simulink model "Motor_La"  (Simulink 7.9)
settings: Solver=ode45  StartTime=0.0  StopTime=0.2  MaxStep=0.0000008  RelTol=1e-8
values from neighbouring files (symbols this model uses):
  J_ges = Jm+Jc/i_getr^2    (= 1.07037741047e-06)    [Sim_Kinematik_Modelle.m]    (also in Tol_Kinematik_Modell.m = Jm+Jc/i_getr^2)
  La = 0*1.792e-3    (= 0)    [DC_Motor_RI_Comp.m]    (also in Sim_Kinematik_Modelle.m = 0.0067; Tol_Kinematik_Modell.m = rnd_vect(n_s,'normal',[La_nom La_tol/3]))
  M_motor = 0.8*M_Load    (= 0.000824029771398)    [DC_Motor_RI_Comp.m]    (also in Sim_Kinematik_Modelle.m = -0.00561973731383; Tol_Kinematik_Modell.m = M_last./(i_getr.*eta_getr))
  Mo = Io*Psi    (= 0.000558650326277)    [DC_Motor_RI_Comp.m]    (also in Sim_Kinematik_Modelle.m = 0.00152232213911; Tol_Kinematik_Modell.m = Io.*Psi)
  Psi = 1/Ispez    (= 0.0159159637116)    [DC_Motor_RI_Comp.m]    (also in Sim_Kinematik_Modelle.m = 0.0173484004456; Tol_Kinematik_Modell.m = Psi_20*(1+Kemf*(T(T_N)-20)))
  Ra = 6.7    [DC_Motor_RI_Comp.m]    (also in Sim_Kinematik_Modelle.m = 5.1322; Tol_Kinematik_Modell.m = Ra_20*(1+Kr*(T(T_N)-20)))
  T_on = linspace(0,0.05,800)    [DC_Motor_RI_Comp.m]    (also in Sim_Kinematik_Modelle.m; Tol_Kinematik_Modell.m = rnd_vect(n_s,'normal',[T_on_nom T_on_tol/3]))
  U_max = U_max_w(i_U)    [DC_Motor_RI_Comp.m]    (also in Sim_Kinematik_Modelle.m; Tol_Kinematik_Modell.m = rnd_vect(n_s,'normal',[U_max_nom U_max_tol/3]))
settings Model: Creator=dep02378  LastModifiedBy=dep02378
settings OptimizationCC: InitFltsAndDblsToZero=on
settings DebuggingCC: FcnCallInpInsideContextMsg=Use local settings  StrictBusMsg=Warning
settings GRTTargetCC: CombineOutputUpdateFcns=off  GRTInterface=on

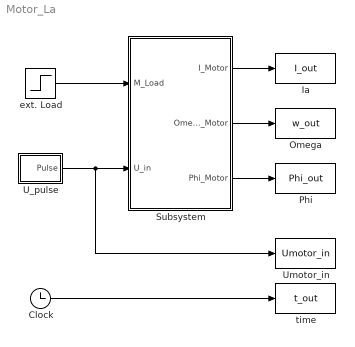
== system Motor_La ==
  Clock : Clock
  Ia : ToWorkspace  VariableName=I_out  SampleTime=-1
  Omega : ToWorkspace  VariableName=w_out  SampleTime=-1
  Phi : ToWorkspace  VariableName=Phi_out  SampleTime=-1
  Subsystem : Subsystem
  U_pulse : Subsystem
  Umotor_in : ToWorkspace  VariableName=Umotor_in  SampleTime=-1
  ext. Load : Step  Time=0  After=M_motor  SampleTime=0
  time : ToWorkspace  VariableName=t_out  SampleTime=-1
  wires:
  Clock/1 -> time/1
  ext. Load/1 -> Subsystem/1(M_Load)
  Subsystem/3(Phi_Motor) -> Phi/1
  U_pulse/1(Pulse) -> Umotor_in/1, Subsystem/2(U_in)
  Subsystem/1(I_Motor) -> Ia/1
  Subsystem/2(Omega_Motor) -> Omega/1

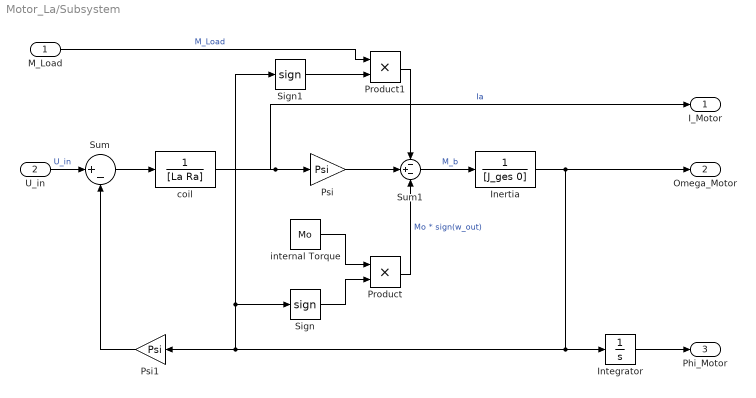
== system Motor_La/Subsystem ==
  M_Load : Inport
  U_in : Inport  Port=2
  Inertia : TransferFcn  Denominator=[J_ges 0]
  Integrator : Integrator
  Product : Product  RndMeth=Zero
  Product1 : Product  RndMeth=Zero
  Psi : Gain  Gain=Psi
  Psi1 : Gain  Gain=Psi
  Sign : Signum  ZeroCross=off
  Sign1 : Signum  ZeroCross=off
  Sum : Sum  Inputs=|+-
  Sum1 : Sum  Inputs=-+-
  coil : TransferFcn  Denominator=[La Ra]
  internal Torque : Constant  Value=Mo
  I_Motor : Outport
  Omega_Motor : Outport  Port=2
  Phi_Motor : Outport  Port=3
  wires:
  Sum/1 -> coil/1
  coil/1 -> Psi/1, I_Motor/1  "Ia"
  Inertia/1 -> Integrator/1, Psi1/1, Sign/1, Sign1/1, Omega_Motor/1
  Sum1/1 -> Inertia/1  "M_b"
  Psi/1 -> Sum1/2
  Product/1 -> Sum1/3  "Mo * sign(w_out)"
  internal Torque/1 -> Product/1
  Sign/1 -> Product/2
  Integrator/1 -> Phi_Motor/1
  Product1/1 -> Sum1/1
  Sign1/1 -> Product1/2
  M_Load/1 -> Product1/1  "M_Load"
  U_in/1 -> Sum/1  "U_in"
  Psi1/1 -> Sum/2

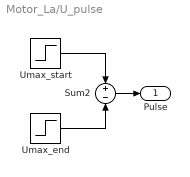
== system Motor_La/U_pulse ==
  Sum2 : Sum  Inputs=+-
  Umax_end : Step  Time=T_on  After=U_max  SampleTime=0
  Umax_start : Step  Time=0  Before=T_on  After=U_max  SampleTime=0
  Pulse : Outport
  wires:
  Umax_end/1 -> Sum2/2
  Umax_start/1 -> Sum2/1
  Sum2/1 -> Pulse/1
